simulink model "System_Architecture_Gera_V1_0"  (R2020a)
settings: Solver=VariableStepAuto  StartTime=0.0  StopTime=10.0  RelTol=1e-3
undefined symbols (not defined in the file): Goal_Location, Map, Start
libraries: robotalgslib x1, robotcorelib x1
settings Model: Creator=user  LastModifiedBy=user

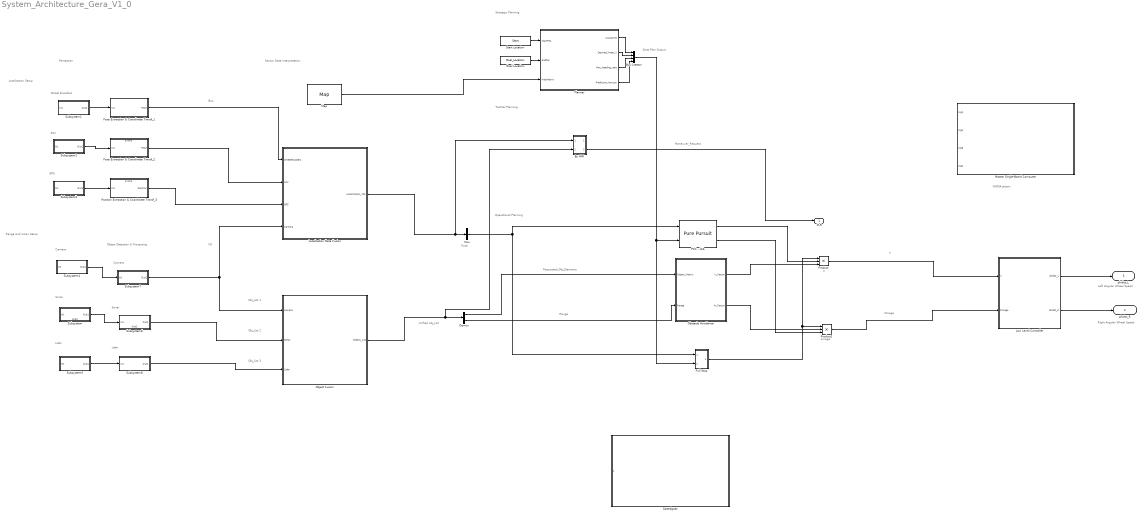
== system System_Architecture_Gera_V1_0 ==
  note: Maneuver_Request
  note: Bus..
  note: Obj_List 1
  note: VO
  note: NVIDIA Jetson
  note: Range
  note: Left Angular Wheel Speed
  note: Omega
  note: V
  note: Pose
  note: Strat.Plan Output
  note: Perception
  note: V
  note: omega
  note: Strategic Planning
  note: Wheel Encoders
  note: Sonar
  note: IMU
  note: GPS
  note: Camera
  note: Localization Setup
  note: Range and Vision Setup
  note: Lidar
  note: Sensor Data Interpretation
  note: Unified obj_List
  note: Right Angular Wheel Speed
  note: Requested_Obj_Elements
  note: Object Detection
      | & Processing
  note: Camera
  note: Lidar
  note: Sonar
  note: Obj_List 2
  note: Obj_List 3
  note: Tactical Planning
  note: Operational Planning
  " Obstacle Avoidance " : MATLAB Function  TreatAsAtomicUnit=on
  Bus Creator : BusCreator  Inputs=4
  By HMI : Subsystem
  Demux : Demux  Outputs=2
  Full Stop : Subsystem
  Goal Location : Constant  Value=Goal_Location
  Localization Data Fusion : MATLAB Function  TreatAsAtomicUnit=on
  Low Level Controller : MATLAB Function  TreatAsAtomicUnit=on
  Map : Constant  Value=Map
  Master Single-Board Computer : MATLAB Function  TreatAsAtomicUnit=on
  Mux : Mux  Inputs=1
  Object Fusion : MATLAB Function  TreatAsAtomicUnit=on
  PFC...LKA : robotalgslib/Pure Pursuit  DesiredLinearVelocity=0.8  MaxAngularVelocity=1  LookaheadDistance=1  TargetDirPort=off  SimulateUsing=Code generation
  Planner : MATLAB Function  TreatAsAtomicUnit=on
  Pose Extraction & Coordinate Transf_1 : Subsystem
  Pose Extraction & Coordinate Transf_2 : Subsystem
  Position Extraction & Coordinate Transf_3 : Subsystem
  Product : Product  Inputs=3
  Product1 : Product  Inputs=3
  "Speedgoat " : MATLAB Function  TreatAsAtomicUnit=on
  Start Location : Constant  Value=Start
  Subsystem : Subsystem
      settings: PortSchema="{\"entries\":[{\"content\":{\"sides\":[{\"content\":{\"connectorIds\":[\"In1\"]},\"type\":\"ConnectorPlacement.EquallySpacedRectSide\",\"uuid\":\"e12de4e3-7626-4c26-8ba2-c587ebf01e53\"},{\"content\":{\"connectorIds\":[\"Out1\"],\"side\":\"RIGHT\"},\"type\":\"ConnectorPlacement.EquallySpacedRectSide\",\"uuid\":\"0359bd44-2cf5-4332-8d76-03b01f15ad87\"},{\"content\":{\"connectorIds\":[],\"side\":\"TOP\"},\"type\":\"ConnectorPlacement.EquallySpacedRectSide\",\"uuid\":\"fe6d17ef-8830-4964-b243-9b4ce9a3f7a6\"},{\"content\":{\"connectorIds\":[\"Out2\"],\"side\":\"BOTTOM\"},\"type\":\"ConnectorPlacement.EquallySpacedRectSide\",\"uuid\":\"c579116e-1f7e-41e7-99df-f35a85b92586\"}]},\"type\":\"ConnectorPlacement.EquallySpacedConnector\",\"uuid\":\"f96e67a7-3827-4941-8ae2-3774148a56ac\"}],\"packageUris\":[\"http://schema.mathworks.com/mf0/Connector/19700101\"],\"version\":\"1.0\"}"
  Subsystem1 : Subsystem
  Subsystem2 : Subsystem
  Subsystem3 : Subsystem
  Subsystem4 : Subsystem
  Subsystem5 : Subsystem
  Subsystem6 : Subsystem
      settings: PortSchema="{\"entries\":[{\"content\":{\"sides\":[{\"content\":{\"connectorIds\":[\"In1\"]},\"type\":\"ConnectorPlacement.EquallySpacedRectSide\",\"uuid\":\"e12de4e3-7626-4c26-8ba2-c587ebf01e53\"},{\"content\":{\"connectorIds\":[\"Out1\"],\"side\":\"RIGHT\"},\"type\":\"ConnectorPlacement.EquallySpacedRectSide\",\"uuid\":\"0359bd44-2cf5-4332-8d76-03b01f15ad87\"},{\"content\":{\"connectorIds\":[],\"side\":\"TOP\"},\"type\":\"ConnectorPlacement.EquallySpacedRectSide\",\"uuid\":\"fe6d17ef-8830-4964-b243-9b4ce9a3f7a6\"},{\"content\":{\"connectorIds\":[\"Out2\"],\"side\":\"BOTTOM\"},\"type\":\"ConnectorPlacement.EquallySpacedRectSide\",\"uuid\":\"c579116e-1f7e-41e7-99df-f35a85b92586\"}]},\"type\":\"ConnectorPlacement.EquallySpacedConnector\",\"uuid\":\"f96e67a7-3827-4941-8ae2-3774148a56ac\"}],\"packageUris\":[\"http://schema.mathworks.com/mf0/Connector/19700101\"],\"version\":\"1.0\"}"
  Subsystem7 : Subsystem
  Subsystem8 : Subsystem
  M-R : Outport
  phidot_R : Outport  Port=2
  phidot_L : Outport  Port=3
  wires:
  Goal Location/1 -> Planner/2(endPos)
  PFC...LKA/1 -> Product/2
  " Obstacle Avoidance "/1(V_Factor) -> Product/3
  PFC...LKA/2 -> Product1/3
  Start Location/1 -> Planner/1(startPos)
  Subsystem5/1(Out1) -> Subsystem8/1(In1)
  " Obstacle Avoidance "/2(W_Factor) -> Product1/2
  Product/1 -> Low Level Controller/1(V)
  Product1/1 -> Low Level Controller/2(Omega)
  Mux/1 -> Full Stop/1(In1), PFC...LKA/1
  Object Fusion/1(Object_List) -> By HMI/2(In2), Demux/1
  Demux/1 -> " Obstacle Avoidance "/1(Object_Matrix)
  Demux/2 -> " Obstacle Avoidance "/2(Range)
  Subsystem1/1(Out1) -> Pose Extraction & Coordinate Transf_1/1(In1)
  Pose Extraction & Coordinate Transf_1/1(Pose) -> Localization Data Fusion/1(WheelEncoders)
  Subsystem2/1(Out1) -> Pose Extraction & Coordinate Transf_2/1(In1)
  Pose Extraction & Coordinate Transf_2/1(Pose) -> Localization Data Fusion/2(IMU)
  Subsystem3/1(Out1) -> Position Extraction & Coordinate Transf_3/1(In1)
  Position Extraction & Coordinate Transf_3/1(Position) -> Localization Data Fusion/3(GPS)
  Subsystem8/1(Out1) -> Object Fusion/3(Lidar)
  Subsystem4/1(Out1) -> Subsystem7/1(In1)
  Subsystem7/1(Out1) -> Localization Data Fusion/4(Camera), Object Fusion/1(camera)
  Subsystem/1(Out1) -> Subsystem6/1(In1)
  Subsystem6/1(Out1) -> Object Fusion/2(Sonar)
  Map/1 -> Planner/3(mapMatrix)
  Planner/1(waypoints) -> Bus Creator/1
  Planner/2(Desired_linear_V) -> Bus Creator/2
  Planner/3(Max_heading_rate) -> Bus Creator/3
  Planner/4(Prediction_horizon) -> Bus Creator/4
  Bus Creator/1 -> Full Stop/2(In2), PFC...LKA/2
  Full Stop/1(gain) -> Product/1, Product1/1
  By HMI/2(M_R) -> M-R/1
  ? -> "Speedgoat "/1(c)
  Localization Data Fusion/1(Localization_info) -> Mux/1, By HMI/1(In1)
  ? -> Master Single-Board Computer/1(sig1)
  ? -> Master Single-Board Computer/2(sig2)
  ? -> Master Single-Board Computer/3(sig3)
  ? -> Master Single-Board Computer/4(sig4)
  Low Level Controller/1(phidot_L) -> phidot_L/1
  Low Level Controller/2(phidot_R) -> phidot_R/1

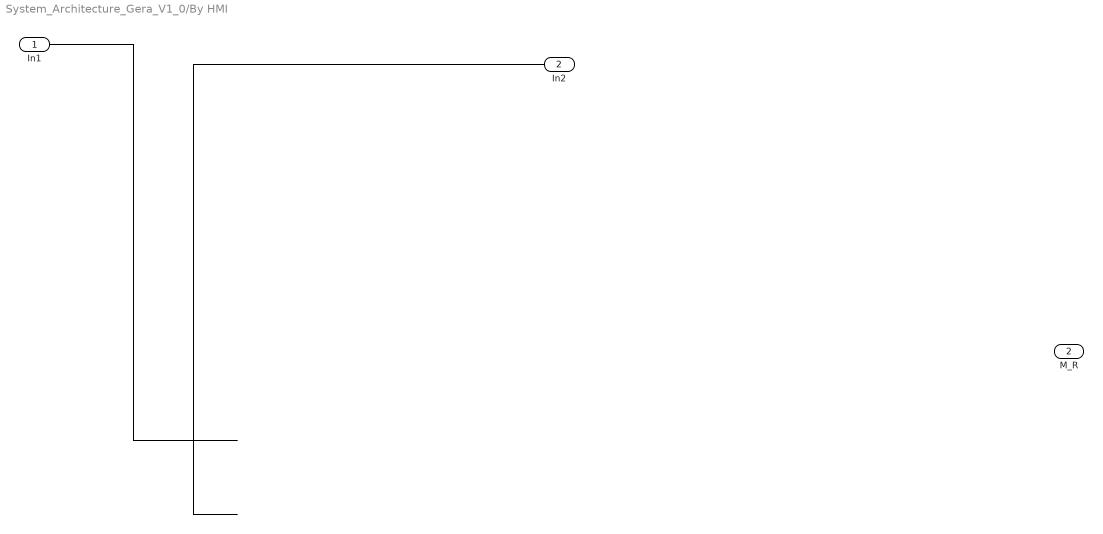
== system System_Architecture_Gera_V1_0/By HMI ==
  In1 : Inport
  In2 : Inport  Port=2
  M_R : Outport  Port=2
  wires:
  ? -> M_R/1
  ? -> ?
  ? -> ?
  In2/1 -> ?
  In1/1 -> ?

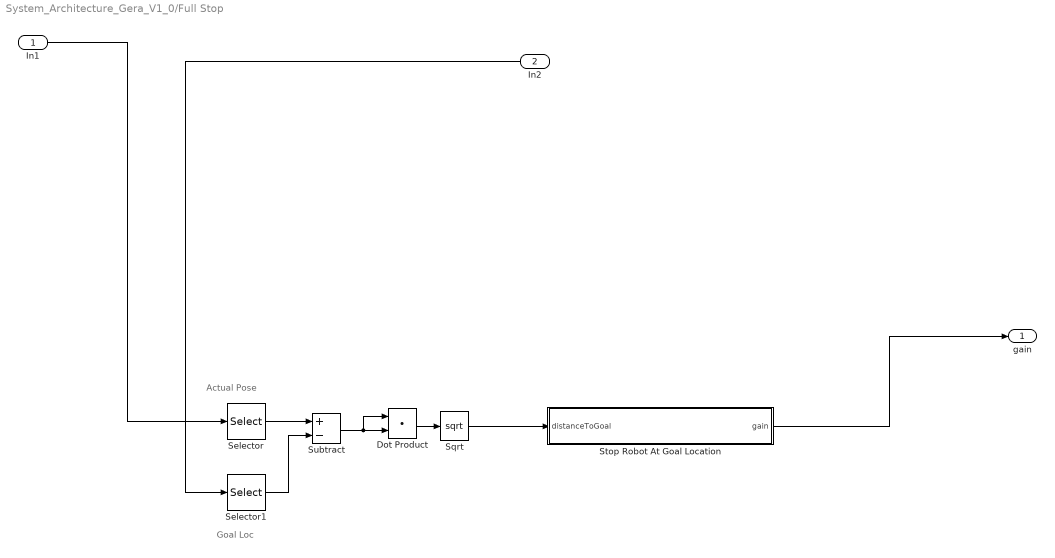
== system System_Architecture_Gera_V1_0/Full Stop ==
  note: Actual Pose
  note: Goal Loc
  In1 : Inport
  In2 : Inport  Port=2
  Dot Product : DotProduct  InputSameDT=on  OutDataTypeStr=Inherit: Inherit via internal rule
  Selector : Selector  InputPortWidth=3  IndexOptions=Index vector (dialog)  Indices=[1 2]  OutputSizes=1
  Selector1 : Selector  InputPortWidth=3  IndexOptions=Index vector (dialog)  Indices=[1 2]  OutputSizes=1
  Sqrt : Sqrt  SaturateOnIntegerOverflow=on
  Stop Robot At Goal Location : MATLAB Function  TreatAsAtomicUnit=on
  Subtract : Sum  Inputs=+-
  gain : Outport
  wires:
  Stop Robot At Goal Location/1(gain) -> gain/1
  Selector/1 -> Subtract/1
  Dot Product/1 -> Sqrt/1
  Sqrt/1 -> Stop Robot At Goal Location/1(distanceToGoal)
  Selector1/1 -> Subtract/2
  Subtract/1 -> Dot Product/1, Dot Product/2
  In2/1 -> Selector1/1
  In1/1 -> Selector/1

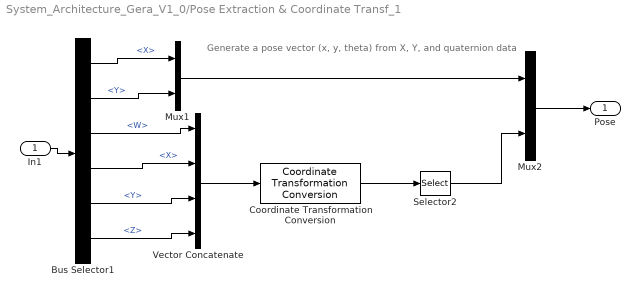
== system System_Architecture_Gera_V1_0/Pose Extraction & Coordinate Transf_1 ==
  note: Generate a pose vector (x, y, theta) from X, Y, and quaternion data
  In1 : Inport
  Bus Selector1 : BusSelector  OutputSignals=Pose.Pose.Position.X,Pose.Pose.Position.Y,Pose.Pose.Orientation.W,Pose.Pose.Orientation.X,Pose.Pose.Orientation.Y,Pose.Pose.Orientation.Z
  Coordinate Transformation Conversion : robotcorelib/Coordinate Transformation Conversion  InputRepresentation=Quaternion  InputEulerSequence=ZYX  ShowTrVecInputPort=on  OutputRepresentation=Euler Angles  OutputEulerSequence=ZYX  ShowTrVecOutputPort=on  SimulateUsing=Interpreted execution
      settings: SourceProductBaseCode=NV,RO,RR
  Mux1 : Mux  Inputs=2
  Mux2 : Mux  Inputs=2
  Selector2 : Selector  InputPortWidth=3  IndexOptions=Index vector (dialog)  Indices=1  OutputSizes=1
  Vector Concatenate : Concatenate  NumInputs=4
  Pose : Outport  VectorParamsAs1DForOutWhenUnconnected=off
  wires:
  Vector Concatenate/1 -> Coordinate Transformation Conversion/1
  Coordinate Transformation Conversion/1 -> Selector2/1
  Mux1/1 -> Mux2/1
  Selector2/1 -> Mux2/2
  Mux2/1 -> Pose/1
  Bus Selector1/6 -> Vector Concatenate/4  "<Z>"
  Bus Selector1/1 -> Mux1/1  "<X>"
  Bus Selector1/4 -> Vector Concatenate/2  "<X>"
  Bus Selector1/2 -> Mux1/2  "<Y>"
  Bus Selector1/5 -> Vector Concatenate/3  "<Y>"
  In1/1 -> Bus Selector1/1
  Bus Selector1/3 -> Vector Concatenate/1  "<W>"

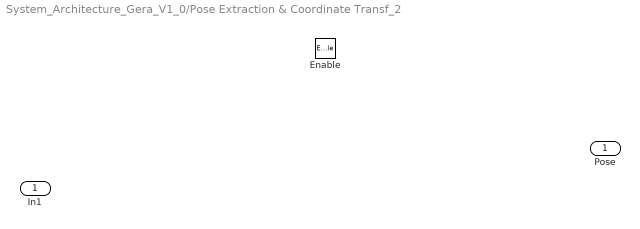
== system System_Architecture_Gera_V1_0/Pose Extraction & Coordinate Transf_2 ==
  In1 : Inport
  Enable : EnablePort
  Pose : Outport  VectorParamsAs1DForOutWhenUnconnected=off

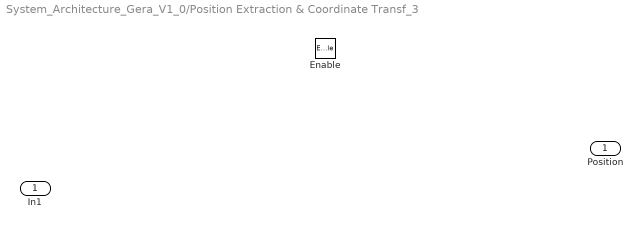
== system System_Architecture_Gera_V1_0/Position Extraction & Coordinate Transf_3 ==
  In1 : Inport
  Enable : EnablePort
  Position : Outport  VectorParamsAs1DForOutWhenUnconnected=off

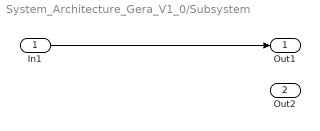
== system System_Architecture_Gera_V1_0/Subsystem ==
  In1 : Inport
  Out1 : Outport
  Out2 : Outport  Port=2
  wires:
  In1/1 -> Out1/1

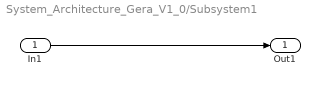
== system System_Architecture_Gera_V1_0/Subsystem1 ==
  In1 : Inport
  Out1 : Outport
  wires:
  In1/1 -> Out1/1

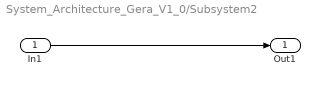
== system System_Architecture_Gera_V1_0/Subsystem2 ==
  In1 : Inport
  Out1 : Outport
  wires:
  In1/1 -> Out1/1

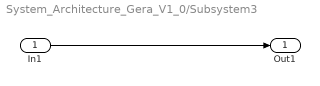
== system System_Architecture_Gera_V1_0/Subsystem3 ==
  In1 : Inport
  Out1 : Outport
  wires:
  In1/1 -> Out1/1

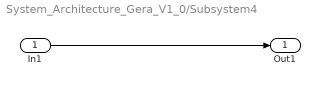
== system System_Architecture_Gera_V1_0/Subsystem4 ==
  In1 : Inport
  Out1 : Outport
  wires:
  In1/1 -> Out1/1

== system System_Architecture_Gera_V1_0/Subsystem5 ==
  In1 : Inport
  Out1 : Outport
  wires:
  In1/1 -> Out1/1

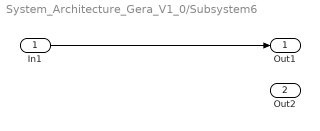
== system System_Architecture_Gera_V1_0/Subsystem6 ==
  In1 : Inport
  Out1 : Outport
  Out2 : Outport  Port=2
  wires:
  In1/1 -> Out1/1

== system System_Architecture_Gera_V1_0/Subsystem7 ==
  In1 : Inport
  Out1 : Outport
  wires:
  In1/1 -> Out1/1

== system System_Architecture_Gera_V1_0/Subsystem8 ==
  In1 : Inport
  Out1 : Outport
  wires:
  In1/1 -> Out1/1

== matlab function System_Architecture_Gera_V1_0/Full Stop/Stop Robot At Goal Location ==
  data: distanceToGoal input; gain output
function gain  = slowDownNearGoal(distanceToGoal)
%%slowDownNearGoal gradually slows the robot when it reaches a goal location.

%continue to move at the normal angular and linear velocity
gain = 1;

%assume that the robot is away from goal
%awayFromGoal = 1;

%threshold to determine if the robot has reached the goal
atGoalThreshold = 0.5;
slowThreshold = 1;

%if the robot is within range and should start slowing down
if(distanceToGoal < slowThreshold)
    
    %speed reduction gain
    gain = distanceToGoal / slowThreshold;
    if(distanceToGoal < atGoalThreshold)
        %stop the robot entirely
        gain = 0;
        %the robot has reached the goal
        %awayFromGoal = 0;
    end
end

== matlab function System_Architecture_Gera_V1_0/Localization Data Fusion ==
  settings: updateMethod=DISCRETE
  data: WheelEncoders input size=[1 2]; IMU input size=[1 2]; Localization_info output size=[100 2]; GPS input; Camera input
function Localization_info = Localization (WheelEncoders, IMU, GPS, Camera)

%fusion for robot's Localization

== matlab function System_Architecture_Gera_V1_0/Planner ==
  settings: updateMethod=DISCRETE
  data: startPos input size=[1 2]; endPos input size=[1 2]; waypoints output size=[100 2]; mapMatrix input; Desired_linear_V output; Max_heading_rate output; Prediction_horizon output
function [waypoints, Desired_linear_V, Max_heading_rate, Prediction_horizon] = planning(startPos, endPos, mapMatrix)

== matlab function System_Architecture_Gera_V1_0/Object Fusion ==
  settings: updateMethod=DISCRETE
  data: camera input size=[1 2]; Sonar input size=[1 2]; Object_List output size=[100 2]; Lidar input
function Object_List  = Objects (camera, Sonar, Lidar)

== matlab function System_Architecture_Gera_V1_0/ Obstacle Avoidance  ==
  data: Object_Matrix input; Range input; V_Factor output size=1; W_Factor output
function [V_Factor, W_Factor] = Obstacle_avoidance(Object_Matrix, Range)

== matlab function System_Architecture_Gera_V1_0/Speedgoat  ==
  data: c input
function Real_Time_impl(c)

== matlab function System_Architecture_Gera_V1_0/Low Level Controller ==
  data: V input; phidot_L output size=1; Omega input; phidot_R output
function [phidot_L, phidot_R]  = LowLevel_Control(V, Omega)

== matlab function System_Architecture_Gera_V1_0/Master Single-Board Computer ==
  data: sig1 input; sig2 input; sig3 input; sig4 input
function Master_Comp(sig1,sig2, sig3, sig4)
